simulink model "test_buildingblocks_newbasicblk_20150723"  (R2014a)
settings: Solver=ode45  StartTime=0.0  StopTime=100  FixedStep=0.001e-3  RelTol=1e-8  AbsTol=1e-11
values from neighbouring files (symbols this model uses):
  A_FB_EN = 1    [test_buildingblocks_newbasicblk_20150723_Sim.m]
  A_FB_EN0 = 1    [test_buildingblocks_newbasicblk_20150723_Sim.m]
  A_FB_EN01 = 0    [test_buildingblocks_newbasicblk_20150723_Sim.m]
  A_FB_EN1 = 1    [test_buildingblocks_newbasicblk_20150723_Sim.m]
  A_FB_EN12 = 0    [test_buildingblocks_newbasicblk_20150723_Sim.m]
  A_FB_EN4 = 0.5    [test_buildingblocks_newbasicblk_20150723_Sim.m]
  A_FB_EN5 = 0    [test_buildingblocks_newbasicblk_20150723_Sim.m]
  A_FB_EN_FI = 0    [test_buildingblocks_newbasicblk_20150723_Sim.m]
  B_FB_EN = 1    [test_buildingblocks_newbasicblk_20150723_Sim.m]
  B_FB_EN0 = 1    [test_buildingblocks_newbasicblk_20150723_Sim.m]
  B_FB_EN01 = 0    [test_buildingblocks_newbasicblk_20150723_Sim.m]
  B_FB_EN1 = 0    [test_buildingblocks_newbasicblk_20150723_Sim.m]
  B_FB_EN11 = 1    [test_buildingblocks_newbasicblk_20150723_Sim.m]
  B_FB_EN12 = 0    [test_buildingblocks_newbasicblk_20150723_Sim.m]
  B_FB_EN_FI = 0    [test_buildingblocks_newbasicblk_20150723_Sim.m]
  C_FF_EN = 1    [test_buildingblocks_newbasicblk_20150723_Sim.m]
  C_FF_ENb = 0    [test_buildingblocks_newbasicblk_20150723_Sim.m]
  D_FF_EN = 1    [test_buildingblocks_newbasicblk_20150723_Sim.m]
  D_FF_EN1 = 1    [test_buildingblocks_newbasicblk_20150723_Sim.m]
  KDfw = 10    [test_buildingblocks_newbasicblk_20150723_Model.m]    (also in test_buildingblocks_newbasicblk_20150723_Sim.m)
  KDfw0 = 10    [test_buildingblocks_newbasicblk_20150723_Sim.m]
  KDfw01 = 5    [test_buildingblocks_newbasicblk_20150723_Model.m]    (also in test_buildingblocks_newbasicblk_20150723_Sim.m)
  KDfw02 = 10    [test_buildingblocks_newbasicblk_20150723_Model.m]    (also in test_buildingblocks_newbasicblk_20150723_Sim.m)
  KDfw03 = 30    [test_buildingblocks_newbasicblk_20150723_Model.m]    (also in test_buildingblocks_newbasicblk_20150723_Sim.m)
  KDfw2 = 10    [test_buildingblocks_newbasicblk_20150723_Sim.m]
  KDrv = 10    [test_buildingblocks_newbasicblk_20150723_Model.m]    (also in test_buildingblocks_newbasicblk_20150723_Sim.m)
  KDrv0 = 10    [test_buildingblocks_newbasicblk_20150723_Sim.m]
  KDrv01 = 10    [test_buildingblocks_newbasicblk_20150723_Model.m]    (also in test_buildingblocks_newbasicblk_20150723_Sim.m)
  KDrv02 = 5    [test_buildingblocks_newbasicblk_20150723_Model.m]    (also in test_buildingblocks_newbasicblk_20150723_Sim.m)
  KDrv03 = 10    [test_buildingblocks_newbasicblk_20150723_Model.m]    (also in test_buildingblocks_newbasicblk_20150723_Sim.m)
  KDrv2 = 10    [test_buildingblocks_newbasicblk_20150723_Sim.m]
  KDrv5 = 10000000    [test_buildingblocks_newbasicblk_20150723_Sim.m]
  KDrv6 = 10000000    [test_buildingblocks_newbasicblk_20150723_Sim.m]
  kr1 = 10*kr_1/KDrv01    (= 10)    [test_buildingblocks_newbasicblk_20150723_Model.m]    (also in test_buildingblocks_newbasicblk_20150723_Sim.m)
  kr11 = 10    [test_buildingblocks_newbasicblk_20150723_Sim.m]
  kr1_01 = 5    [test_buildingblocks_newbasicblk_20150723_Sim.m]
  kr2 = 10*kr_1/KDrv02    (= 20)    [test_buildingblocks_newbasicblk_20150723_Model.m]    (also in test_buildingblocks_newbasicblk_20150723_Sim.m = 5)
  kr22 = 5    [test_buildingblocks_newbasicblk_20150723_Sim.m]
  krC = 10    [test_buildingblocks_newbasicblk_20150723_Sim.m]
  krC4 = 20    [test_buildingblocks_newbasicblk_20150723_Sim.m]
  krD = 10    [test_buildingblocks_newbasicblk_20150723_Sim.m]
  n = 1    [test_buildingblocks_newbasicblk_20150723_Sim.m]
  ratC = 0    [test_buildingblocks_newbasicblk_20150723_Sim.m]
  ratC0 = 0    [test_buildingblocks_newbasicblk_20150723_Sim.m]
  ratC01 = 1    [test_buildingblocks_newbasicblk_20150723_Sim.m]
  ratC02 = 0.1    [test_buildingblocks_newbasicblk_20150723_Sim.m]
  ratC03 = 2    [test_buildingblocks_newbasicblk_20150723_Sim.m]
  ratC04 = 0.5    [test_buildingblocks_newbasicblk_20150723_Sim.m]
  ratC05 = 10    [test_buildingblocks_newbasicblk_20150723_Sim.m]
  ratC10 = 0.06    [test_buildingblocks_newbasicblk_20150723_Model.m]    (also in test_buildingblocks_newbasicblk_20150723_Sim.m = 0.6)
  ratC11 = 0.2    [test_buildingblocks_newbasicblk_20150723_Sim.m]
  ratC12 = 0.2    [test_buildingblocks_newbasicblk_20150723_Model.m]    (also in test_buildingblocks_newbasicblk_20150723_Sim.m = 1)
  ratC13 = 0.2    [test_buildingblocks_newbasicblk_20150723_Model.m]    (also in test_buildingblocks_newbasicblk_20150723_Sim.m = 2)
  ratC14 = 0.3    [test_buildingblocks_newbasicblk_20150723_Model.m]    (also in test_buildingblocks_newbasicblk_20150723_Sim.m = 3)
  ratC15 = 0.2    [test_buildingblocks_newbasicblk_20150723_Model.m]    (also in test_buildingblocks_newbasicblk_20150723_Sim.m = 10)
  ratC4 = 1    [test_buildingblocks_newbasicblk_20150723_Model.m]    (also in test_buildingblocks_newbasicblk_20150723_Sim.m)
  ratC5 = 3    [test_buildingblocks_newbasicblk_20150723_Model.m]    (also in test_buildingblocks_newbasicblk_20150723_Sim.m)
  ratC7 = 1    [test_buildingblocks_newbasicblk_20150723_Model.m]    (also in test_buildingblocks_newbasicblk_20150723_Sim.m = 2)
  ratC8 = 0.1    [test_buildingblocks_newbasicblk_20150723_Model.m]    (also in test_buildingblocks_newbasicblk_20150723_Sim.m)
  ratC9 = 0.03    [test_buildingblocks_newbasicblk_20150723_Model.m]    (also in test_buildingblocks_newbasicblk_20150723_Sim.m = 0)
  ratD = 0    [test_buildingblocks_newbasicblk_20150723_Sim.m]
(part 3 of 3)

== system test_buildingblocks_newbasicblk_20150723/NEW_BASIC7 ==
  In1 : Inport
  In9 : Inport  Port=2
  In6 : Inport  Port=3
  In7 : Inport  Port=4
  In4 : Inport  Port=5
  In5 : Inport  Port=6
  In2 : Inport  Port=7
  In8 : Inport  Port=8
  In3 : Inport  Port=9
  A_FB_EN sw : Gain  Gain=A_FB_EN5
  Add1 : Sum  Inputs=-+
  Add{2..3,9..10} (4 alike) : Sum  Inputs=+-
  Add{4..6,8,11} (5 alike) : Sum
  Add7 : Sum  Inputs=-+
  B_FB_EN sw : Gain  Gain=B_FB_EN1
  Exponential : Fcn  Expr=u(1)^n
  FF_EN sw{,3..5} (4 alike) : Gain  Gain=C_FF_EN
  FF_EN sw1 : Gain  Gain=C_FF_ENb
  FF_EN sw2 : Gain  Gain=C_FF_ENb
  Gain1 : Gain  Gain=1/KDfw
  Gain2 : Gain  Gain=kr1
  Gain3 : Gain  Gain=kr2
  Gain4 : Gain  Gain=1/KDrv
  Gain5 : Gain
  Gain6 : Gain
  Gain7 : Gain  Gain=ratC9
  Integrator1 : Integrator
  Manual Switch : ManualSwitch  CurrentSetting=0
  Product1 : Product  RndMeth=Zero
  Product2 : Product  RndMeth=Zero
  Out1 : Outport
  Out4 : Outport  Port=2
  Out2 : Outport  Port=3
  Out3 : Outport  Port=4
  Out5 : Outport  Port=5
  Out6 : Outport  Port=6
  Out7 : Outport  Port=7
  Out8 : Outport  Port=8
  Out9 : Outport  Port=9
  Out10 : Outport  Port=10
  Out11 : Outport  Port=11
  Out13 : Outport  Port=12
  wires:
  FF_EN sw5/1 -> Add3/2
  FF_EN sw4/1 -> Add11/2
  Add11/1 -> Add3/1
  Gain3/1 -> Add10/2
  Gain2/1 -> Add10/1
  Add10/1 -> Integrator1/1
  Add8/1 -> Out4/1  "Dtot"
  In8/1 -> Add8/2  "Ddeg"
  In2/1 -> Add8/1  "Dprod"
  Gain7/1 -> Add6/1
  Add5/1 -> Out8/1  "rate_rv_tot"
  Add6/1 -> Add9/1, Add5/2, Gain3/1
  FF_EN sw2/1 -> Add9/2
  FF_EN sw3/1 -> Add5/1
  Gain4/1 -> Out6/1, FF_EN sw2/1, FF_EN sw3/1, FF_EN sw5/1  "rate_rv"
  Gain6/1 -> Out11/1  "Cfree_copy"
  Product2/1 -> Gain4/1
  In7/1 -> Gain5/1, Product2/2  "Dfree"
  In6/1 -> Gain7/1, Product2/1, Gain6/1  "Cfree"
  In5/1 -> Add6/2  "Cdeg"
  FF_EN sw1/1 -> Add7/1
  Manual Switch/1 -> Out1/1, A_FB_EN sw/1, B_FB_EN sw/1  "Ctot"
  Integrator1/1 -> Manual Switch/2
  In3/1 -> Manual Switch/1  "Ctot_in"
  Add9/1 -> Out10/1  "rate_rv_up"
  Add7/1 -> Out9/1  "rate_fw_up"
  FF_EN sw/1 -> Add4/2
  Add4/1 -> Out7/1  "rate_fw_tot"
  In4/1 -> Add7/2, Add4/1, Add11/1  "Cprod"
  Product1/1 -> FF_EN sw1/1, FF_EN sw4/1, FF_EN sw/1, Out5/1  "rate_fw"
  Exponential/1 -> Product1/2
  Gain1/1 -> Exponential/1
  In9/1 -> Add2/1  "Btot"
  In1/1 -> Add1/2  "Atot"
  Add1/1 -> Product1/1, Out2/1  "Afree"
  Add2/1 -> Out3/1, Gain1/1  "Bfree"
  Add3/1 -> Gain2/1
  A_FB_EN sw/1 -> Add1/1
  B_FB_EN sw/1 -> Add2/2
  Gain5/1 -> Out13/1  "Dfree_copy"

== system test_buildingblocks_newbasicblk_20150723/NEW_BASIC8 ==
  In1 : Inport
  In9 : Inport  Port=2
  In6 : Inport  Port=3
  In7 : Inport  Port=4
  In4 : Inport  Port=5
  In5 : Inport  Port=6
  In2 : Inport  Port=7
  In8 : Inport  Port=8
  In3 : Inport  Port=9
  A_FB_EN sw : Gain  Gain=A_FB_EN1
  Add1 : Sum  Inputs=-+
  Add{2..3,9..10} (4 alike) : Sum  Inputs=+-
  Add{4..6,8,11} (5 alike) : Sum
  Add7 : Sum  Inputs=-+
  B_FB_EN sw : Gain  Gain=B_FB_EN
  Exponential : Fcn  Expr=u(1)^n
  FF_EN sw{,3..5} (4 alike) : Gain  Gain=C_FF_EN
  FF_EN sw1 : Gain  Gain=C_FF_ENb
  FF_EN sw2 : Gain  Gain=C_FF_ENb
  Gain1 : Gain  Gain=1/KDfw
  Gain2 : Gain  Gain=kr1
  Gain3 : Gain  Gain=kr2
  Gain4 : Gain  Gain=1/KDrv
  Gain5 : Gain
  Gain6 : Gain
  Gain7 : Gain  Gain=ratC11
  Integrator1 : Integrator
  Manual Switch : ManualSwitch  CurrentSetting=0
  Product1 : Product  RndMeth=Zero
  Product2 : Product  RndMeth=Zero
  Out1 : Outport
  Out4 : Outport  Port=2
  Out2 : Outport  Port=3
  Out3 : Outport  Port=4
  Out5 : Outport  Port=5
  Out6 : Outport  Port=6
  Out7 : Outport  Port=7
  Out8 : Outport  Port=8
  Out9 : Outport  Port=9
  Out10 : Outport  Port=10
  Out11 : Outport  Port=11
  Out13 : Outport  Port=12
  wires:
  Gain5/1 -> Out13/1  "Dfree_copy"
  B_FB_EN sw/1 -> Add2/2
  A_FB_EN sw/1 -> Add1/1
  Add3/1 -> Gain2/1
  Add2/1 -> Gain1/1, Out3/1  "Bfree"
  Add1/1 -> Out2/1, Product1/1  "Afree"
  In1/1 -> Add1/2  "Atot"
  In9/1 -> Add2/1  "Btot"
  Gain1/1 -> Exponential/1
  Exponential/1 -> Product1/2
  Product1/1 -> Out5/1, FF_EN sw/1, FF_EN sw4/1, FF_EN sw1/1  "rate_fw"
  In4/1 -> Add11/1, Add4/1, Add7/2  "Cprod"
  Add4/1 -> Out7/1  "rate_fw_tot"
  FF_EN sw/1 -> Add4/2
  Add7/1 -> Out9/1  "rate_fw_up"
  Add9/1 -> Out10/1  "rate_rv_up"
  In3/1 -> Manual Switch/1  "Ctot_in"
  Integrator1/1 -> Manual Switch/2
  Manual Switch/1 -> B_FB_EN sw/1, A_FB_EN sw/1, Out1/1  "Ctot"
  FF_EN sw1/1 -> Add7/1
  In5/1 -> Add6/2  "Cdeg"
  In6/1 -> Gain6/1, Product2/1, Gain7/1  "Cfree"
  In7/1 -> Product2/2, Gain5/1  "Dfree"
  Product2/1 -> Gain4/1
  Gain6/1 -> Out11/1  "Cfree_copy"
  Gain4/1 -> FF_EN sw5/1, FF_EN sw3/1, FF_EN sw2/1, Out6/1  "rate_rv"
  FF_EN sw3/1 -> Add5/1
  FF_EN sw2/1 -> Add9/2
  Add6/1 -> Gain3/1, Add5/2, Add9/1
  Add5/1 -> Out8/1  "rate_rv_tot"
  Gain7/1 -> Add6/1
  In2/1 -> Add8/1  "Dprod"
  In8/1 -> Add8/2  "Ddeg"
  Add8/1 -> Out4/1  "Dtot"
  Add10/1 -> Integrator1/1
  Gain2/1 -> Add10/1
  Gain3/1 -> Add10/2
  Add11/1 -> Add3/1
  FF_EN sw4/1 -> Add11/2
  FF_EN sw5/1 -> Add3/2

== system test_buildingblocks_newbasicblk_20150723/NEW_BASIC9 ==
  In1 : Inport
  In9 : Inport  Port=2
  In6 : Inport  Port=3
  In7 : Inport  Port=4
  In4 : Inport  Port=5
  In5 : Inport  Port=6
  In2 : Inport  Port=7
  In8 : Inport  Port=8
  In3 : Inport  Port=9
  A_FB_EN sw : Gain  Gain=A_FB_EN5
  Add1 : Sum  Inputs=-+
  Add{2..3,9..10} (4 alike) : Sum  Inputs=+-
  Add{4..6,8,11} (5 alike) : Sum
  Add7 : Sum  Inputs=-+
  B_FB_EN sw : Gain  Gain=B_FB_EN1
  Exponential : Fcn  Expr=u(1)^n
  FF_EN sw{,3..5} (4 alike) : Gain  Gain=C_FF_EN
  FF_EN sw1 : Gain  Gain=C_FF_ENb
  FF_EN sw2 : Gain  Gain=C_FF_ENb
  Gain1 : Gain  Gain=1/KDfw
  Gain2 : Gain  Gain=kr1
  Gain3 : Gain  Gain=kr2
  Gain4 : Gain  Gain=1/KDrv
  Gain5 : Gain
  Gain6 : Gain
  Gain7 : Gain  Gain=ratC10
  Integrator1 : Integrator
  Manual Switch : ManualSwitch  CurrentSetting=0
  Product1 : Product  RndMeth=Zero
  Product2 : Product  RndMeth=Zero
  Out1 : Outport
  Out4 : Outport  Port=2
  Out2 : Outport  Port=3
  Out3 : Outport  Port=4
  Out5 : Outport  Port=5
  Out6 : Outport  Port=6
  Out7 : Outport  Port=7
  Out8 : Outport  Port=8
  Out9 : Outport  Port=9
  Out10 : Outport  Port=10
  Out11 : Outport  Port=11
  Out13 : Outport  Port=12
  wires:
  FF_EN sw5/1 -> Add3/2
  FF_EN sw4/1 -> Add11/2
  Add11/1 -> Add3/1
  Gain3/1 -> Add10/2
  Gain2/1 -> Add10/1
  Add10/1 -> Integrator1/1
  Add8/1 -> Out4/1  "Dtot"
  In8/1 -> Add8/2  "Ddeg"
  In2/1 -> Add8/1  "Dprod"
  Gain7/1 -> Add6/1
  Add5/1 -> Out8/1  "rate_rv_tot"
  Add6/1 -> Add9/1, Add5/2, Gain3/1
  FF_EN sw2/1 -> Add9/2
  FF_EN sw3/1 -> Add5/1
  Gain4/1 -> Out6/1, FF_EN sw2/1, FF_EN sw3/1, FF_EN sw5/1  "rate_rv"
  Gain6/1 -> Out11/1  "Cfree_copy"
  Product2/1 -> Gain4/1
  In7/1 -> Gain5/1, Product2/2  "Dfree"
  In6/1 -> Gain7/1, Product2/1, Gain6/1  "Cfree"
  In5/1 -> Add6/2  "Cdeg"
  FF_EN sw1/1 -> Add7/1
  Manual Switch/1 -> Out1/1, A_FB_EN sw/1, B_FB_EN sw/1  "Ctot"
  Integrator1/1 -> Manual Switch/2
  In3/1 -> Manual Switch/1  "Ctot_in"
  Add9/1 -> Out10/1  "rate_rv_up"
  Add7/1 -> Out9/1  "rate_fw_up"
  FF_EN sw/1 -> Add4/2
  Add4/1 -> Out7/1  "rate_fw_tot"
  In4/1 -> Add7/2, Add4/1, Add11/1  "Cprod"
  Product1/1 -> FF_EN sw1/1, FF_EN sw4/1, FF_EN sw/1, Out5/1  "rate_fw"
  Exponential/1 -> Product1/2
  Gain1/1 -> Exponential/1
  In9/1 -> Add2/1  "Btot"
  In1/1 -> Add1/2  "Atot"
  Add1/1 -> Product1/1, Out2/1  "Afree"
  Add2/1 -> Out3/1, Gain1/1  "Bfree"
  Add3/1 -> Gain2/1
  A_FB_EN sw/1 -> Add1/1
  B_FB_EN sw/1 -> Add2/2
  Gain5/1 -> Out13/1  "Dfree_copy"
